simulink model "modelagem_2021a_2"  (R2021a)
settings: Solver=ode4  StartTime=0.0  StopTime=3  FixedStep=10^-5  MaxStep=10^-6  RelTol=1e-3
StopFcn:
  | q = out.logsout{2}.Values;
  | wc = out.logsout{1}.Values;
  | r = find(out.logsout,"r")
  | r = r.Values;
  | r=r.Data;
  | eul = find(out.logsout,"eul");
  | eul = eul.Values.Data;
  | norma = find(out.logsout,"n");
  | norma = norma.Values.Data;
  | qL = find(out.logsout,"qL");
  | qL = qL.Values.Data;
  | t = q.Time;
  | figure(1)
  | plot(t,eul);
  | legend('$\psi$','$\theta$','$\phi$','Interpreter','latex')
  | xlabel("Tempo [s]")
  | ylabel("Ângulos de Euler [°]")
  | title("Ângulos de Euler ZYZ do Cubli")
  | 
  | figure(2)
  | plot(q.Time,q.Data,q.Time,qL)
  | legend("q0","q1","q2","q3","q0 Linear","q1 Linear","q2 Linear","q3 Linear")
  | ylabel("Quaternions")
  | xlabel("Tempo [s]")
  | title("Quaternions do Cubli - Posição Angular")
  | hold off
  | 
  | figure(3)
  | plot(wc.Time,wc.Data)
  | legend("\omega_x","\omega_y","\omega_z")
  | ylabel("Velocidade Angular [rad/s]")
  | xlabel("Tempo [s]")
  | title("Velocidade Angular do Cubli")
  | figure(4)
  | plot3(r(:,1),r(:,2),r(:,3),'-o')
  | xlabel('X [m]')
  | ylabel('Y [m]')
  | zlabel('Z [m]')
  | axis([-0.1 0.1 -0.1 0.1 0 0.2])
  | title('Trajetória do Centro de Massa')
  | figure(5)
  | plot(t,norma)
  | xlabel("Norma do quaternion");
  | ylabel("Tempo [s]")
  | title("Norma do quaternion do Cubli durante simulação numérica")
values from neighbouring files (symbols this model uses):
  A = [0	0	0	0.5	0	0 ... (first row only)    [ITAE.m]    (also in Itae_control.m; classic_control.m = [0., 0., 0., 0.5, 0., 0.; control_techniques.m = [0., 0., 0., 0.5, 0., 0.; controlabilidade_observabilidade.m = [0., 0., 0., 0.5, 0., 0.)
  b = 17.03*10^(-6)    (= 1.703e-05)    [controle_script.m]    (also in modelagem_script.m)
  B = [0	0	0 ... (first row only)    [ITAE.m]    (also in Itae_control.m; classic_control.m = [0.	0.	0.; control_techniques.m = [0.	0.	0.; controlabilidade_observabilidade.m = [0.	0.	0.)
  C = tf([Kd,Kp,Ki],[1,0])    [ITAE.m]    (also in Itae_control.m = [1	0	0	0	0	0; classic_control.m = [1	0	0	0	0	0; control_techniques.m = [1	0	0	0	0	0; controlabilidade_observabilidade.m = [1	0	0	0	0	0)
  D = zeros(3,3)    [ITAE.m]    (also in Itae_control.m; classic_control.m; control_techniques.m = zeros(6,3); controlabilidade_observabilidade.m)
  g = [0;0;-9.81]    [controle_script.m]    (also in modelagem_script.m)
  Ic = [0.01008 -0.00309375 -0.00309375 ... (first row only)    [modelagem_script.m]
  Ic_inv = inv(Ic)    [controle_script.m]    (also in modelagem_script.m)
  Ic_p = [v(2) 0 0 ; 0 v(3) 0 ; 0 0 v(1)]    [modelagem_script.m]
  Ic_pinv = inv(Ic_p)    [modelagem_script.m]
  mc = 0.55    [controle_script.m]    (also in modelagem_script.m)
  q00 = [cos(phi_p/2);e*sin(phi_p/2)]    [controle_script.m]    (also in modelagem_script.m = [cos(phi_u/2);e_u*sin(phi_u/2)])
  q00_p = [1;0;0;0]    [modelagem_script.m]
  rc = [0;0;norm([0.0954545, 0.0954545, 0.0954545])]    [controle_script.m]    (also in modelagem_script.m = [0.0954545;0.0954545;0.0954545])
  rc_p = [0;0;norm(rc)]    [modelagem_script.m]
  Tau = [0;0;0]    [modelagem_script.m]
  w00 = [0.1;0.1;0.1]    [controle_script.m]    (also in modelagem_script.m = 2*pi/sqrt(3)*[1;1;1])
  w00_p = [0;0;0]    [modelagem_script.m]
libraries: vrlib x5, aerolibutil x1
settings Model: Creator=guimi  LastModifiedBy=lucap
settings SolverCC: InitialStep=10^-6
settings DataIOCC: SaveFinalState=on  InspectSignalLogs=on
settings DebuggingCC: UnconnectedInputMsg=none  UnconnectedOutputMsg=none  UnconnectedLineMsg=none
settings ModelReferenceCC: EnableRefExpFcnMdlSchedulingChecks=off
settings RTWCC: Description=Generic Real-Time Target  DLArmComputeVersion=20.02.1

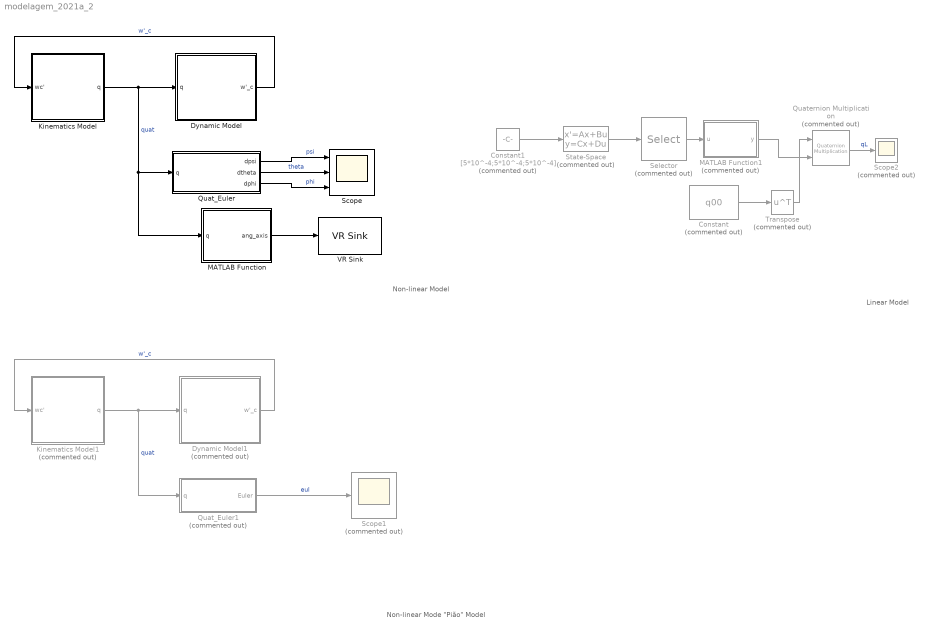
== system modelagem_2021a_2 ==
  note: Non-linear Model
  note: Non-linear Mode
      | "Pião" Model
  note: Linear Model
  Constant : Constant  Commented=on  Value=q00
  Constant1 : Constant  Commented=on  Value=[5*10^-4;5*10^-4;5*10^-4]
  Dynamic Model : Subsystem
  Dynamic Model1 : Subsystem  Commented=on
  Kinematics Model : Subsystem
  Kinematics Model1 : Subsystem  Commented=on
  MATLAB Function : MATLAB Function  TreatAsAtomicUnit=on
  MATLAB Function1 : MATLAB Function  Commented=on  TreatAsAtomicUnit=on
  Quat_Euler : Subsystem
  Quat_Euler1 : Subsystem  Commented=on
  Quaternion Multiplication : aerolibutil/Quaternion Multiplication  Commented=on
  Scope : Scope  NumInputPorts=3
  Scope1 : Scope  Commented=on
  Scope2 : Scope  Commented=on
  Selector : Selector  Commented=on  InputPortWidth=6  IndexOptions=Index vector (dialog)  Indices=[1 2 3]  OutputSizes=1
  State-Space : StateSpace  Commented=on  A=A  B=B  C=C  D=D  InitialCondition=[0;0;0;0;0;0]
  Transpose : Math  Commented=on  Operator=transpose  SaturateOnIntegerOverflow=on
  VR Sink : vrlib/VR Sink  InstantiateOnLoad=on  SampleTime=0.01  ViewEnable=on  RemoteChange=off  RemoteView=on  FieldsWritten=Cubli.rotation.4.1.1.double  WorldFileName=Cubo.x3d  WorldDescription=Cubo  AutoView=on  VideoDimensions=[550 700]  AllowVariableSize=off
  wires:
  Kinematics Model/1(q) -> MATLAB Function/1(q), Quat_Euler/1(q), Dynamic Model/1(q)  "quat"
  Dynamic Model/1(w'_c) -> Kinematics Model/1(wc')  "w'_c"
  MATLAB Function/1(ang_axis) -> VR Sink/1
  Quat_Euler/2(dtheta) -> Scope/2  "theta"
  Quat_Euler/3(dphi) -> Scope/3  "phi"
  Quat_Euler/1(dpsi) -> Scope/1  "psi"
  Kinematics Model1/1(q) -> Quat_Euler1/1(q), Dynamic Model1/1(q)  "quat"
  Dynamic Model1/1(w'_c) -> Kinematics Model1/1(wc')  "w'_c"
  Quat_Euler1/1(Euler) -> Scope1/1  "eul"
  MATLAB Function1/1(y) -> Quaternion Multiplication/2
  State-Space/1 -> Selector/1
  Transpose/1 -> Quaternion Multiplication/1
  Quaternion Multiplication/1 -> Scope2/1  "qL"
  Constant/1 -> Transpose/1
  Selector/1 -> MATLAB Function1/1(u)
  Constant1/1 -> State-Space/1

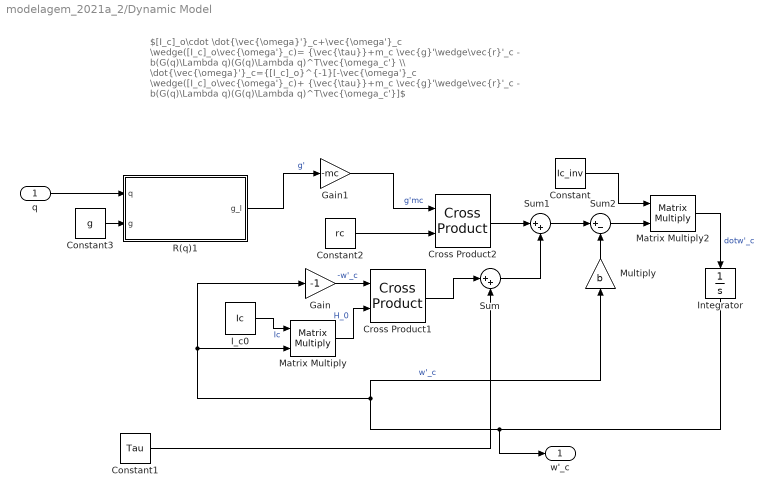
== system modelagem_2021a_2/Dynamic Model ==
  note: $[I_c]_o\cdot \dot{\vec{\omega}'}_c+\vec{\omega'}_c \wedge([I_c]_o\vec{\omega'}_c)= {\vec{\tau}}+m_c \vec{g}'\wedge\vec{r}'_c - b(G(q)\Lambda q)(G(q)\Lambda q)^T\vec{\omega_c'} \\ \dot{\vec{\omega}'}_c={[I_c]_o}^{-1}[-\vec{\omega'}_c \wedge([I_c]_o\vec{\omega'}_c)+ {\vec{\tau}}+m_c \vec{g}'\wedge\vec{r}'_c - b(G(q)\Lambda q)(G(q)\Lambda q)^T\vec{\omega_c'}]$
  q : Inport
  Constant : Constant  Value=Ic_inv
  Constant1 : Constant  Value=Tau
  Constant2 : Constant  Value=rc
  Constant3 : Constant  Value=g
  Cross Product1 : vrlib/Utilities/Cross Product
  Cross Product2 : vrlib/Utilities/Cross Product
  Gain : Gain  Gain=-1
  Gain1 : Gain  Gain=-mc
  I_c0 : Constant  Value=Ic
  Integrator : Integrator  InitialCondition=w00
  Matrix Multiply : Product  Multiplication=Matrix(*)
  Matrix Multiply2 : Product  Multiplication=Matrix(*)
  Multiply : Gain  Gain=b
  R(q)1 : MATLAB Function  TreatAsAtomicUnit=on
  Sum : Sum  Inputs=|++
  Sum1 : Sum  Inputs=|++
  Sum2 : Sum  Inputs=|+-
  w'_c : Outport
  wires:
  I_c0/1 -> Matrix Multiply/1  "Ic"
  Integrator/1 -> w'_c/1, Gain/1, Matrix Multiply/2, Multiply/1  "w'_c"
  Matrix Multiply/1 -> Cross Product1/2  "H_0"
  Gain/1 -> Cross Product1/1  "-w'_c"
  Cross Product1/1 -> Sum/1
  q/1 -> R(q)1/1(q)
  Gain1/1 -> Cross Product2/1  "g'mc"
  Constant2/1 -> Cross Product2/2
  Sum/1 -> Sum1/2
  Sum1/1 -> Sum2/1
  Multiply/1 -> Sum2/2
  Sum2/1 -> Matrix Multiply2/2
  Constant/1 -> Matrix Multiply2/1
  Matrix Multiply2/1 -> Integrator/1  "dotw'_c"
  Cross Product2/1 -> Sum1/1
  R(q)1/1(g_l) -> Gain1/1  "g'"
  Constant3/1 -> R(q)1/2(g)
  Constant1/1 -> Sum/2

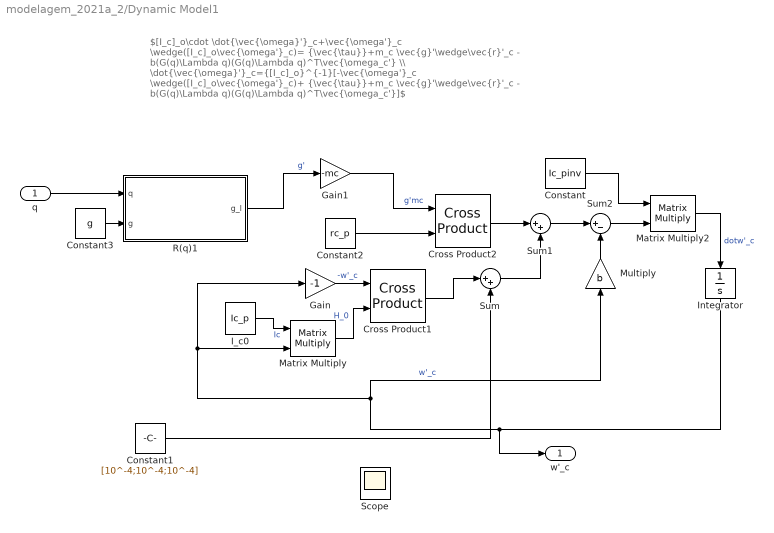
== system modelagem_2021a_2/Dynamic Model1 ==
  note: $[I_c]_o\cdot \dot{\vec{\omega}'}_c+\vec{\omega'}_c \wedge([I_c]_o\vec{\omega'}_c)= {\vec{\tau}}+m_c \vec{g}'\wedge\vec{r}'_c - b(G(q)\Lambda q)(G(q)\Lambda q)^T\vec{\omega_c'} \\ \dot{\vec{\omega}'}_c={[I_c]_o}^{-1}[-\vec{\omega'}_c \wedge([I_c]_o\vec{\omega'}_c)+ {\vec{\tau}}+m_c \vec{g}'\wedge\vec{r}'_c - b(G(q)\Lambda q)(G(q)\Lambda q)^T\vec{\omega_c'}]$
  q : Inport
  Constant : Constant  Value=Ic_pinv
  Constant1 : Constant  Value=[10^-4;10^-4;10^-4]
  Constant2 : Constant  Value=rc_p
  Constant3 : Constant  Value=g
  Cross Product1 : vrlib/Utilities/Cross Product
  Cross Product2 : vrlib/Utilities/Cross Product
  Gain : Gain  Gain=-1
  Gain1 : Gain  Gain=-mc
  I_c0 : Constant  Value=Ic_p
  Integrator : Integrator  InitialCondition=w00_p
  Matrix Multiply : Product  Multiplication=Matrix(*)
  Matrix Multiply2 : Product  Multiplication=Matrix(*)
  Multiply : Gain  Gain=b
  R(q)1 : MATLAB Function  TreatAsAtomicUnit=on
  Scope : Scope
  Sum : Sum  Inputs=|++
  Sum1 : Sum  Inputs=|++
  Sum2 : Sum  Inputs=|+-
  w'_c : Outport
  wires:
  I_c0/1 -> Matrix Multiply/1  "Ic"
  Integrator/1 -> w'_c/1, Gain/1, Matrix Multiply/2, Multiply/1  "w'_c"
  Matrix Multiply/1 -> Cross Product1/2  "H_0"
  Gain/1 -> Cross Product1/1  "-w'_c"
  Cross Product1/1 -> Sum/1
  q/1 -> R(q)1/1(q)
  Gain1/1 -> Cross Product2/1  "g'mc"
  Constant2/1 -> Cross Product2/2
  Sum/1 -> Sum1/2
  Sum1/1 -> Sum2/1
  Multiply/1 -> Sum2/2
  Sum2/1 -> Matrix Multiply2/2
  Constant/1 -> Matrix Multiply2/1
  Matrix Multiply2/1 -> Integrator/1  "dotw'_c"
  Cross Product2/1 -> Sum1/1
  R(q)1/1(g_l) -> Gain1/1  "g'"
  Constant3/1 -> R(q)1/2(g)
  Constant1/1 -> Sum/2

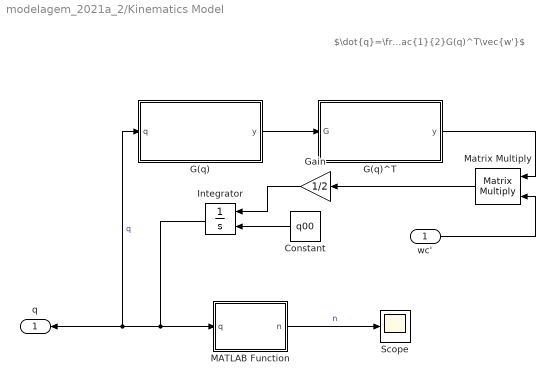
== system modelagem_2021a_2/Kinematics Model ==
  note: $\dot{q}=\frac{1}{2}G(q)^T\vec{w'}$
  wc' : Inport
  Constant : Constant  Value=q00
  G(q) : MATLAB Function  TreatAsAtomicUnit=on
  G(q)^T : MATLAB Function  TreatAsAtomicUnit=on
  Gain : Gain  Gain=1/2
  Integrator : Integrator  InitialConditionSource=external  InitialCondition=q00  UpperSaturationLimit=1  LowerSaturationLimit=-1
  MATLAB Function : MATLAB Function  TreatAsAtomicUnit=on
  Matrix Multiply : Product  Multiplication=Matrix(*)
  Scope : Scope
  q : Outport
  wires:
  G(q)/1(y) -> G(q)^T/1(G)
  wc'/1 -> Matrix Multiply/2
  G(q)^T/1(y) -> Matrix Multiply/1
  Integrator/1 -> MATLAB Function/1(q), G(q)/1(q), q/1  "q"
  Matrix Multiply/1 -> Gain/1
  Constant/1 -> Integrator/2
  Gain/1 -> Integrator/1
  MATLAB Function/1(n) -> Scope/1  "n"

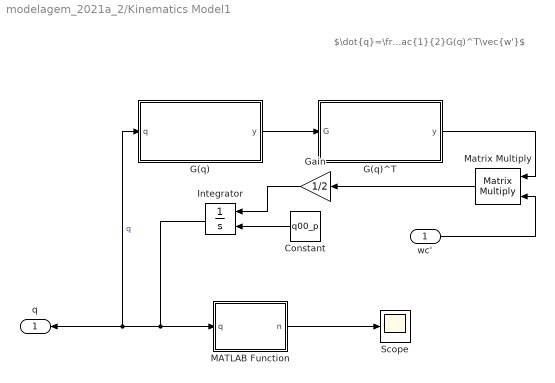
== system modelagem_2021a_2/Kinematics Model1 ==
  note: $\dot{q}=\frac{1}{2}G(q)^T\vec{w'}$
  wc' : Inport
  Constant : Constant  Value=q00_p
  G(q) : MATLAB Function  TreatAsAtomicUnit=on
  G(q)^T : MATLAB Function  TreatAsAtomicUnit=on
  Gain : Gain  Gain=1/2
  Integrator : Integrator  InitialConditionSource=external  InitialCondition=q00  UpperSaturationLimit=1  LowerSaturationLimit=-1
  MATLAB Function : MATLAB Function  TreatAsAtomicUnit=on
  Matrix Multiply : Product  Multiplication=Matrix(*)
  Scope : Scope
  q : Outport
  wires:
  G(q)/1(y) -> G(q)^T/1(G)
  wc'/1 -> Matrix Multiply/2
  G(q)^T/1(y) -> Matrix Multiply/1
  Integrator/1 -> MATLAB Function/1(q), G(q)/1(q), q/1  "q"
  Matrix Multiply/1 -> Gain/1
  Constant/1 -> Integrator/2
  Gain/1 -> Integrator/1
  MATLAB Function/1(n) -> Scope/1

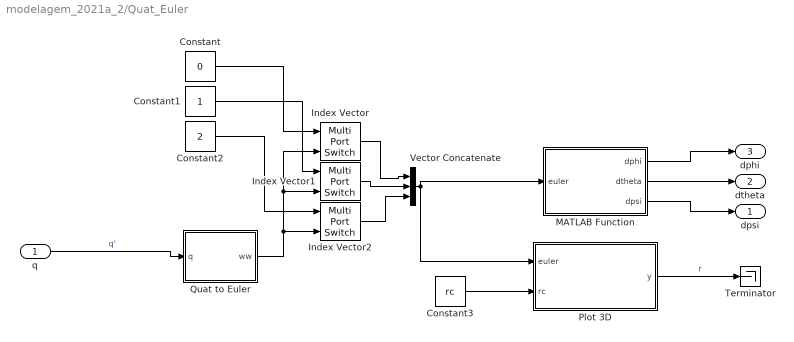
== system modelagem_2021a_2/Quat_Euler ==
  q : Inport
  Constant : Constant  Value=0
  Constant1 : Constant
  Constant2 : Constant  Value=2
  Constant3 : Constant  Value=rc
  Index Vector : MultiPortSwitch  DataPortOrder=Zero-based contiguous  Inputs=1  zeroidx=on
  Index Vector1 : MultiPortSwitch  DataPortOrder=Zero-based contiguous  Inputs=1  zeroidx=on
  Index Vector2 : MultiPortSwitch  DataPortOrder=Zero-based contiguous  Inputs=1  zeroidx=on
  MATLAB Function : MATLAB Function  TreatAsAtomicUnit=on
  Plot 3D : MATLAB Function  TreatAsAtomicUnit=on
  Quat to Euler : MATLAB Function  TreatAsAtomicUnit=on
  Terminator : Terminator
  Vector Concatenate : Concatenate  NumInputs=3
  dpsi : Outport
  dtheta : Outport  Port=2
  dphi : Outport  Port=3
  wires:
  Quat to Euler/1(ww) -> Index Vector/2, Index Vector1/2, Index Vector2/2
  Constant2/1 -> Index Vector2/1
  Constant1/1 -> Index Vector1/1
  Constant/1 -> Index Vector/1
  MATLAB Function/2(dtheta) -> dtheta/1
  q/1 -> Quat to Euler/1(q)  "q'"
  MATLAB Function/3(dpsi) -> dpsi/1
  MATLAB Function/1(dphi) -> dphi/1
  Index Vector/1 -> Vector Concatenate/1
  Index Vector1/1 -> Vector Concatenate/2
  Index Vector2/1 -> Vector Concatenate/3
  Vector Concatenate/1 -> Plot 3D/1(euler), MATLAB Function/1(euler)
  Plot 3D/1(y) -> Terminator/1  "r"
  Constant3/1 -> Plot 3D/2(rc)

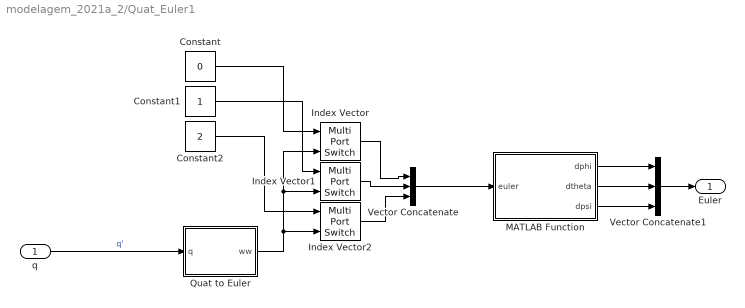
== system modelagem_2021a_2/Quat_Euler1 ==
  q : Inport
  Constant : Constant  Value=0
  Constant1 : Constant
  Constant2 : Constant  Value=2
  Index Vector : MultiPortSwitch  DataPortOrder=Zero-based contiguous  Inputs=1  zeroidx=on
  Index Vector1 : MultiPortSwitch  DataPortOrder=Zero-based contiguous  Inputs=1  zeroidx=on
  Index Vector2 : MultiPortSwitch  DataPortOrder=Zero-based contiguous  Inputs=1  zeroidx=on
  MATLAB Function : MATLAB Function  TreatAsAtomicUnit=on
  Quat to Euler : MATLAB Function  TreatAsAtomicUnit=on
  Vector Concatenate : Concatenate  NumInputs=3
  Vector Concatenate1 : Concatenate  NumInputs=3
  Euler : Outport
  wires:
  Quat to Euler/1(ww) -> Index Vector/2, Index Vector1/2, Index Vector2/2
  Constant2/1 -> Index Vector2/1
  Constant1/1 -> Index Vector1/1
  Constant/1 -> Index Vector/1
  MATLAB Function/2(dtheta) -> Vector Concatenate1/2
  q/1 -> Quat to Euler/1(q)  "q'"
  MATLAB Function/3(dpsi) -> Vector Concatenate1/3
  MATLAB Function/1(dphi) -> Vector Concatenate1/1
  Index Vector/1 -> Vector Concatenate/1
  Index Vector1/1 -> Vector Concatenate/2
  Index Vector2/1 -> Vector Concatenate/3
  Vector Concatenate/1 -> MATLAB Function/1(euler)
  Vector Concatenate1/1 -> Euler/1

== matlab function modelagem_2021a_2/MATLAB Function1 ==
  data: u input; y output
function y = fcn(u)

y = [sqrt(1-u(1)^2 - u(2)^2 - u(3)^2),u(1),u(2),u(3)];

== matlab function modelagem_2021a_2/Quat_Euler1/MATLAB Function ==
  data: dphi output; dtheta output; euler input; dpsi output
function [dphi,dtheta,dpsi] = fcn(euler)


dpsi = 180/pi *euler(3);
dtheta = 180/pi *euler(2);
dphi = 180/pi *euler(1);
end

== matlab function modelagem_2021a_2/Quat_Euler1/Quat to Euler ==
  data: q input; ww output
     function ww = fcn(q)

[a,angles] = quat2eul(q.','ZYZ');
ww = angles.';

% w = [psi;theteul;phi];

== matlab function modelagem_2021a_2/Dynamic Model/R(q)1 ==
  data: q input; g_l output; g input
function g_l = fcn(q,g)
    I = eye(3);
    qi = [q(2);q(3);q(4)];
    qT = qi.';
    g_l = 2*dot(qi,g)*qi + q(1)^2*g + 2*q(1)*cross(g,qi) - dot(qi,qi)*g;
end

== matlab function modelagem_2021a_2/Quat_Euler/MATLAB Function ==
  data: dphi output; dtheta output; euler input; dpsi output
function [dphi,dtheta,dpsi] = fcn(euler)


dpsi = 180/pi *euler(3);
dtheta = 180/pi *euler(2);
dphi = 180/pi *euler(1);
end

== matlab function modelagem_2021a_2/Quat_Euler/Quat to Euler ==
  data: q input; ww output
     function ww = fcn(q)

angles = quat2eul(q.','ZYZ');
ww = angles.';

% w = [psi;theteul;phi];

== matlab function modelagem_2021a_2/Kinematics Model/MATLAB Function ==
  data: q input; n output
function n = norm(q)
    n = sqrt(q(1)^2+q(2)^2+q(3)^2+q(4)^2);

== matlab function modelagem_2021a_2/Kinematics Model/G(q) ==
  data: q input; y output
function y = fcn(q)
    y = [-q(2) q(1) q(4) -q(3); -q(3) -q(4) q(1) q(2); -q(4) q(3) -q(2) q(1)];  
end

== matlab function modelagem_2021a_2/Kinematics Model/G(q)^T ==
  data: G input; y output
function y = fcn(G)
    y = G.';  
end

== matlab function modelagem_2021a_2/MATLAB Function ==
  data: q input; ang_axis output
function ang_axis = fcn(q)

angle = 2*acos(q(1));
x = q(2)/sqrt(1 - q(1)^2);
y = q(3)/sqrt(1 - q(1)^2);
z = q(4)/sqrt(1 - q(1)^2);
ang_axis = [x,y,z,angle];

== matlab function modelagem_2021a_2/Dynamic Model1/R(q)1 ==
  data: q input; g_l output; g input
function g_l = fcn(q,g)
    I = eye(3);
    qi = [q(2);q(3);q(4)];
    qT = qi.';
    g_l = 2*dot(qi,g)*qi + q(1)^2*g + 2*q(1)*cross(g,qi) - dot(qi,qi)*g;
end

== matlab function modelagem_2021a_2/Quat_Euler/Plot 3D ==
  data: euler input; y output; rc input
function y = fcn(euler,rc)

R1 = [[cos(euler(1)) sin(euler(1)) 0];
      [-sin(euler(1)) cos(euler(1)) 0];
      [0 0 1]];
R2 = [[cos(euler(2)) 0 -sin(euler(2))];
     [0 1 0];
     [sin(euler(2)) 0 cos(euler(2))]];
R3 = [[cos(euler(3)) sin(euler(3)) 0];
      [-sin(euler(3)) cos(euler(3)) 0];
      [0 0 1]];
R = R3*R2*R1;

y =inv(R)*rc;

== matlab function modelagem_2021a_2/Kinematics Model1/G(q) ==
  data: q input; y output
function y = fcn(q)
    y = [-q(2) q(1) q(4) -q(3); -q(3) -q(4) q(1) q(2); -q(4) q(3) -q(2) q(1)];  
end

== matlab function modelagem_2021a_2/Kinematics Model1/G(q)^T ==
  data: G input; y output
function y = fcn(G)
    y = G.';  
end

== matlab function modelagem_2021a_2/Kinematics Model1/MATLAB Function ==
  data: q input; n output
function n = norm(q)
    n = sqrt(q(1)^2+q(2)^2+q(3)^2+q(4)^2);
